simulink model "SPMSMSensorless"  (R2019b)
settings: Solver=VariableStepAuto  StartTime=0.0  StopTime=10  RelTol=1e-3
undefined symbols (not defined in the file): BmRated, DiscIntNeverNeededParam, etaFSO, etaPsiFSO, JmRated, K_dead, kFSO, KiId, KiIq, KiSpd, KpId, KpIq, kPsiFSO, KpSpd, LdRated, LqRated, OutCur_LowerLimit, OutCur_UpperLimit, OutSpd_LowerLimit, OutSpd_UpperLimit, PhiPMRated, Pn, RsRated, SetSpd_n, TsimCurLoop, TsimMotor, UdcRated, V_dead
libraries: simulink x3, eeTransforms x1, powerlib x1
(part 2 of 2)

== system SPMSMSensorless/PWM INT/FSO_RsInf/Clark Transformation4 ==
  U : Inport
  V : Inport  Port=2
  W : Inport  Port=3
  Add : Sum  Inputs=+--
  Add1 : Sum  Inputs=+-
  Gain : Gain  Gain=0.5
  Gain1 : Gain  Gain=0.5
  Gain2 : Gain  Gain=2/3
  Gain3 : Gain  Gain=2/3*0.86602540
  Alpha : Outport
  Beta : Outport  Port=2
  wires:
  Gain3/1 -> Beta/1
  Add1/1 -> Gain3/1
  Gain2/1 -> Alpha/1
  Add/1 -> Gain2/1
  U/1 -> Add/1
  Gain1/1 -> Add/3
  W/1 -> Gain1/1, Add1/2
  Gain/1 -> Add/2
  V/1 -> Gain/1, Add1/1

== system SPMSMSensorless/PWM INT/FSO_RsInf/PLL ==
  Eal : Inport
  Ebe : Inport  Port=2
  Add : Sum  Inputs=+-
  Cos : Trigonometry  Operator=cos
  Discrete-Time Integrator : DiscreteIntegrator  SampleTime=-1  ICPrevOutput=DiscIntNeverNeededParam  ICPrevScaledInput=DiscIntNeverNeededParam
  PID Controller : simulink/Continuous/PID Controller  Controller=PI  Form=Parallel  TimeDomain=Discrete-time  SampleTime=-1  IntegratorMethod=Forward Euler  FilterMethod=Forward Euler  ControllerParametersSource=internal  P=2*10*2*pi  I=(10*2*pi)^2  D=0  UseFilter=on  N=100  TunerSelectOption=Transfer Function Based (PID Tuner App)  InitialConditionSource=internal  InitialConditionForIntegrator=SetSpd_n*5/60*2*pi  InitialConditionForFilter=0  DifferentiatorICPrevScaledInput=0  ExternalReset=none  TrackingMode=off  Kt=1  LimitOutput=off  UpperSaturationLimit=inf  LowerSaturationLimit=-inf  LinearizeAsGain=on  AntiWindupMode=none  Kb=1  POutMin=[]  POutMax=[]  IOutMin=[]  IOutMax=[]  DOutMin=[]  DOutMax=[]  NOutMin=[]  NOutMax=[]  SumOutMin=[]  SumOutMax=[]  SaturationOutMin=[]  SaturationOutMax=[]  PParamMin=[]  PParamMax=[]  IParamMin=[]  IParamMax=[]  DParamMin=[]  DParamMax=[]  NParamMin=[]  NParamMax=[]  KbParamMin=[]  KbParamMax=[]  KtParamMin=[]  KtParamMax=[]  KbOutMin=[]  KbOutMax=[]  KtOutMin=[]  KtOutMax=[]  IntegratorOutMin=[]  IntegratorOutMax=[]  FilterOutMin=[]  FilterOutMax=[]  SumI1OutMin=[]  SumI1OutMax=[]  SumI2OutMin=[]  SumI2OutMax=[]  SumI3OutMin=[]  SumI3OutMax=[]  SumI4OutMin=[]  SumI4OutMax=[]  SumDOutMin=[]  SumDOutMax=[]  DifferentiatorOutMin=[]  DifferentiatorOutMax=[]  FilterDiffOutCoefMin=[]  FilterDiffOutCoefMax=[]  ReciprocalOutMin=[]  ReciprocalOutMax=[]  SumDenOutMin=[]  SumDenOutMax=[]  SumNumOutMin=[]  SumNumOutMax=[]  DivideOutMin=[]  DivideOutMax=[]  IntegratorContinuousStateAttributes=''  IntegratorStateMustResolveToSignalObject=off  IntegratorRTWStateStorageClass=Auto  FilterContinuousStateAttributes=''  FilterStateMustResolveToSignalObject=off  FilterRTWStateStorageClass=Auto  ParallelPVariant=InternalParameters  IdealPVariant=Disabled  IVariant=InternalParameters  DVariant=Disabled  IntegratorVariant=Discrete  SatVariant=Disabled  AWVariant=Passthrough  PCopyVariant=Disabled  TRVariant=Disabled  FdbkBlocksVariant=Forward  IdealPFdbkVariant=Disabled  SatFdbkVariant=Disabled  DerivativeFilterVariant=Disabled  NVariant=Disabled  NCopyVariant=Disabled_SignalSpec  FilterICVariant=Disabled  IntegratorICVariant=InternalICs  ExternalResetVariant=Disabled  TRSumVariant=Passthrough  SumFdbkVariant=Disabled  SumVariant=Sum_PI
  Product : Product
  Product1 : Product
  Sin : Trigonometry
  Unit Delay2 : UnitDelay  SampleTime=-1  HasFrameUpgradeWarning=on
  Unit Delay3 : UnitDelay  SampleTime=-1  HasFrameUpgradeWarning=on
  OmegaE : Outport
  ThetaE : Outport  Port=2
  wires:
  Sin/1 -> Product1/2
  Eal/1 -> Product/1
  Discrete-Time Integrator/1 -> ThetaE/1, Unit Delay3/1, Unit Delay2/1
  Unit Delay2/1 -> Cos/1
  Unit Delay3/1 -> Sin/1
  Product1/1 -> Add/2
  Product/1 -> Add/1
  Cos/1 -> Product/2
  Add/1 -> PID Controller/1
  Ebe/1 -> Product1/1
  PID Controller/1 -> Discrete-Time Integrator/1, OmegaE/1

== system SPMSMSensorless/PWM INT/FSO_RsInfPLL/Clark Transformation3 ==
  U : Inport
  V : Inport  Port=2
  W : Inport  Port=3
  Add : Sum  Inputs=+--
  Add1 : Sum  Inputs=+-
  Gain : Gain  Gain=0.5
  Gain1 : Gain  Gain=0.5
  Gain2 : Gain  Gain=2/3
  Gain3 : Gain  Gain=2/3*0.86602540
  Alpha : Outport
  Beta : Outport  Port=2
  wires:
  V/1 -> Add1/1, Gain/1
  Gain/1 -> Add/2
  W/1 -> Add1/2, Gain1/1
  Gain1/1 -> Add/3
  U/1 -> Add/1
  Add/1 -> Gain2/1
  Gain2/1 -> Alpha/1
  Add1/1 -> Gain3/1
  Gain3/1 -> Beta/1

== system SPMSMSensorless/PWM INT/FSO_RsInfPLL/Clark Transformation4 ==
  U : Inport
  V : Inport  Port=2
  W : Inport  Port=3
  Add : Sum  Inputs=+--
  Add1 : Sum  Inputs=+-
  Gain : Gain  Gain=0.5
  Gain1 : Gain  Gain=0.5
  Gain2 : Gain  Gain=2/3
  Gain3 : Gain  Gain=2/3*0.86602540
  Alpha : Outport
  Beta : Outport  Port=2
  wires:
  V/1 -> Add1/1, Gain/1
  Gain/1 -> Add/2
  W/1 -> Add1/2, Gain1/1
  Gain1/1 -> Add/3
  U/1 -> Add/1
  Add/1 -> Gain2/1
  Gain2/1 -> Alpha/1
  Add1/1 -> Gain3/1
  Gain3/1 -> Beta/1

== system SPMSMSensorless/PWM INT/FSO_RsInfPLL/LPF ==
  In1 : Inport
  Add1 : Sum
  Gain1 : Gain  Gain=1-0.1
  Gain3 : Gain  Gain=0.1
  Unit Delay1 : UnitDelay  SampleTime=-1  HasFrameUpgradeWarning=on
  Out1 : Outport
  wires:
  Add1/1 -> Out1/1, Unit Delay1/1
  Gain1/1 -> Add1/2
  Unit Delay1/1 -> Gain1/1
  Gain3/1 -> Add1/1
  In1/1 -> Gain3/1

== system SPMSMSensorless/PWM INT/FSO_RsInfPLL/PLL ==
  Eal : Inport
  Ebe : Inport  Port=2
  Add : Sum  Inputs=+-
  Cos : Trigonometry  Operator=cos
  Discrete-Time Integrator : DiscreteIntegrator  SampleTime=-1  ICPrevOutput=DiscIntNeverNeededParam  ICPrevScaledInput=DiscIntNeverNeededParam
  Gain1 : Gain  Gain=-1
  PID Controller : simulink/Continuous/PID Controller  Controller=PI  Form=Parallel  TimeDomain=Discrete-time  SampleTime=-1  IntegratorMethod=Forward Euler  FilterMethod=Forward Euler  ControllerParametersSource=internal  P=2*10*2*pi  I=(10*2*pi)^2  D=0  UseFilter=on  N=100  TunerSelectOption=Transfer Function Based (PID Tuner App)  InitialConditionSource=internal  InitialConditionForIntegrator=SetSpd_n*5/60*2*pi  InitialConditionForFilter=0  DifferentiatorICPrevScaledInput=0  ExternalReset=none  TrackingMode=off  Kt=1  LimitOutput=off  UpperSaturationLimit=inf  LowerSaturationLimit=-inf  LinearizeAsGain=on  AntiWindupMode=none  Kb=1  POutMin=[]  POutMax=[]  IOutMin=[]  IOutMax=[]  DOutMin=[]  DOutMax=[]  NOutMin=[]  NOutMax=[]  SumOutMin=[]  SumOutMax=[]  SaturationOutMin=[]  SaturationOutMax=[]  PParamMin=[]  PParamMax=[]  IParamMin=[]  IParamMax=[]  DParamMin=[]  DParamMax=[]  NParamMin=[]  NParamMax=[]  KbParamMin=[]  KbParamMax=[]  KtParamMin=[]  KtParamMax=[]  KbOutMin=[]  KbOutMax=[]  KtOutMin=[]  KtOutMax=[]  IntegratorOutMin=[]  IntegratorOutMax=[]  FilterOutMin=[]  FilterOutMax=[]  SumI1OutMin=[]  SumI1OutMax=[]  SumI2OutMin=[]  SumI2OutMax=[]  SumI3OutMin=[]  SumI3OutMax=[]  SumI4OutMin=[]  SumI4OutMax=[]  SumDOutMin=[]  SumDOutMax=[]  DifferentiatorOutMin=[]  DifferentiatorOutMax=[]  FilterDiffOutCoefMin=[]  FilterDiffOutCoefMax=[]  ReciprocalOutMin=[]  ReciprocalOutMax=[]  SumDenOutMin=[]  SumDenOutMax=[]  SumNumOutMin=[]  SumNumOutMax=[]  DivideOutMin=[]  DivideOutMax=[]  IntegratorContinuousStateAttributes=''  IntegratorStateMustResolveToSignalObject=off  IntegratorRTWStateStorageClass=Auto  FilterContinuousStateAttributes=''  FilterStateMustResolveToSignalObject=off  FilterRTWStateStorageClass=Auto  ParallelPVariant=InternalParameters  IdealPVariant=Disabled  IVariant=InternalParameters  DVariant=Disabled  IntegratorVariant=Discrete  SatVariant=Disabled  AWVariant=Passthrough  PCopyVariant=Disabled  TRVariant=Disabled  FdbkBlocksVariant=Forward  IdealPFdbkVariant=Disabled  SatFdbkVariant=Disabled  DerivativeFilterVariant=Disabled  NVariant=Disabled  NCopyVariant=Disabled_SignalSpec  FilterICVariant=Disabled  IntegratorICVariant=InternalICs  ExternalResetVariant=Disabled  TRSumVariant=Passthrough  SumFdbkVariant=Disabled  SumVariant=Sum_PI
  Product : Product
  Product1 : Product
  Sin : Trigonometry
  Unit Delay2 : UnitDelay  SampleTime=-1  HasFrameUpgradeWarning=on
  Unit Delay3 : UnitDelay  SampleTime=-1  HasFrameUpgradeWarning=on
  OmegaE : Outport
  ThetaE : Outport  Port=2
  wires:
  Sin/1 -> Product1/2
  Gain1/1 -> Product/1
  Discrete-Time Integrator/1 -> ThetaE/1, Unit Delay3/1, Unit Delay2/1
  Unit Delay2/1 -> Cos/1
  Unit Delay3/1 -> Sin/1
  Product1/1 -> Add/2
  Product/1 -> Add/1
  Cos/1 -> Product/2
  Add/1 -> PID Controller/1
  Ebe/1 -> Product1/1
  Eal/1 -> Gain1/1
  PID Controller/1 -> Discrete-Time Integrator/1, OmegaE/1

== system SPMSMSensorless/PWM INT/PsiFSO/Clark Transformation3 ==
  U : Inport
  V : Inport  Port=2
  W : Inport  Port=3
  Add : Sum  Inputs=+--
  Add1 : Sum  Inputs=+-
  Gain : Gain  Gain=0.5
  Gain1 : Gain  Gain=0.5
  Gain2 : Gain  Gain=2/3
  Gain3 : Gain  Gain=2/3*0.86602540
  Alpha : Outport
  Beta : Outport  Port=2
  wires:
  Gain3/1 -> Beta/1
  Add1/1 -> Gain3/1
  Gain2/1 -> Alpha/1
  Add/1 -> Gain2/1
  U/1 -> Add/1
  Gain1/1 -> Add/3
  W/1 -> Gain1/1, Add1/2
  Gain/1 -> Add/2
  V/1 -> Gain/1, Add1/1

== system SPMSMSensorless/PWM INT/PsiFSO/Clark Transformation4 ==
  U : Inport
  V : Inport  Port=2
  W : Inport  Port=3
  Add : Sum  Inputs=+--
  Add1 : Sum  Inputs=+-
  Gain : Gain  Gain=0.5
  Gain1 : Gain  Gain=0.5
  Gain2 : Gain  Gain=2/3
  Gain3 : Gain  Gain=2/3*0.86602540
  Alpha : Outport
  Beta : Outport  Port=2
  wires:
  Gain3/1 -> Beta/1
  Add1/1 -> Gain3/1
  Gain2/1 -> Alpha/1
  Add/1 -> Gain2/1
  U/1 -> Add/1
  Gain1/1 -> Add/3
  W/1 -> Gain1/1, Add1/2
  Gain/1 -> Add/2
  V/1 -> Gain/1, Add1/1

== system SPMSMSensorless/PWM INT/PsiFSORsAD/Clark Transformation3 ==
  U : Inport
  V : Inport  Port=2
  W : Inport  Port=3
  Add : Sum  Inputs=+--
  Add1 : Sum  Inputs=+-
  Gain : Gain  Gain=0.5
  Gain1 : Gain  Gain=0.5
  Gain2 : Gain  Gain=2/3
  Gain3 : Gain  Gain=2/3*0.86602540
  Alpha : Outport
  Beta : Outport  Port=2
  wires:
  V/1 -> Add1/1, Gain/1
  Gain/1 -> Add/2
  W/1 -> Add1/2, Gain1/1
  Gain1/1 -> Add/3
  U/1 -> Add/1
  Add/1 -> Gain2/1
  Gain2/1 -> Alpha/1
  Add1/1 -> Gain3/1
  Gain3/1 -> Beta/1

== system SPMSMSensorless/PWM INT/PsiFSORsAD/Clark Transformation4 ==
  U : Inport
  V : Inport  Port=2
  W : Inport  Port=3
  Add : Sum  Inputs=+--
  Add1 : Sum  Inputs=+-
  Gain : Gain  Gain=0.5
  Gain1 : Gain  Gain=0.5
  Gain2 : Gain  Gain=2/3
  Gain3 : Gain  Gain=2/3*0.86602540
  Alpha : Outport
  Beta : Outport  Port=2
  wires:
  V/1 -> Add1/1, Gain/1
  Gain/1 -> Add/2
  W/1 -> Add1/2, Gain1/1
  Gain1/1 -> Add/3
  U/1 -> Add/1
  Add/1 -> Gain2/1
  Gain2/1 -> Alpha/1
  Add1/1 -> Gain3/1
  Gain3/1 -> Beta/1

== system SPMSMSensorless/PWM INT/PsiFSORsInf/Clark Transformation3 ==
  U : Inport
  V : Inport  Port=2
  W : Inport  Port=3
  Add : Sum  Inputs=+--
  Add1 : Sum  Inputs=+-
  Gain : Gain  Gain=0.5
  Gain1 : Gain  Gain=0.5
  Gain2 : Gain  Gain=2/3
  Gain3 : Gain  Gain=2/3*0.86602540
  Alpha : Outport
  Beta : Outport  Port=2
  wires:
  V/1 -> Add1/1, Gain/1
  Gain/1 -> Add/2
  W/1 -> Add1/2, Gain1/1
  Gain1/1 -> Add/3
  U/1 -> Add/1
  Add/1 -> Gain2/1
  Gain2/1 -> Alpha/1
  Add1/1 -> Gain3/1
  Gain3/1 -> Beta/1

== system SPMSMSensorless/PWM INT/PsiFSORsInf/Clark Transformation4 ==
  U : Inport
  V : Inport  Port=2
  W : Inport  Port=3
  Add : Sum  Inputs=+--
  Add1 : Sum  Inputs=+-
  Gain : Gain  Gain=0.5
  Gain1 : Gain  Gain=0.5
  Gain2 : Gain  Gain=2/3
  Gain3 : Gain  Gain=2/3*0.86602540
  Alpha : Outport
  Beta : Outport  Port=2
  wires:
  V/1 -> Add1/1, Gain/1
  Gain/1 -> Add/2
  W/1 -> Add1/2, Gain1/1
  Gain1/1 -> Add/3
  U/1 -> Add/1
  Add/1 -> Gain2/1
  Gain2/1 -> Alpha/1
  Add1/1 -> Gain3/1
  Gain3/1 -> Beta/1

== system SPMSMSensorless/PWM INT/RealVoltageCompesation /Clark Transformation ==
  U : Inport
  V : Inport  Port=2
  W : Inport  Port=3
  Add : Sum  Inputs=+--
  Add1 : Sum  Inputs=+-
  Gain : Gain  Gain=0.5
  Gain1 : Gain  Gain=0.5
  Gain2 : Gain  Gain=2/3
  Gain3 : Gain  Gain=2/3*0.86602540
  Alpha : Outport
  Beta : Outport  Port=2
  wires:
  V/1 -> Add1/1, Gain/1
  Gain/1 -> Add/2
  W/1 -> Add1/2, Gain1/1
  Gain1/1 -> Add/3
  U/1 -> Add/1
  Add/1 -> Gain2/1
  Gain2/1 -> Alpha/1
  Add1/1 -> Gain3/1
  Gain3/1 -> Beta/1

== system SPMSMSensorless/PWM INT/RealVoltageCompesation /Park Transformation ==
  Alpha : Inport
  Beta : Inport  Port=2
  theta : Inport  Port=3
  Add : Sum
  Add1 : Sum  Inputs=+-
  Product{,1..3} (4 alike) : Product
  Sin : Trigonometry  OutputSignalType=real
  Sin1 : Trigonometry  Operator=cos  OutputSignalType=real
  D : Outport
  Q : Outport  Port=2
  wires:
  Product/1 -> Add/1
  Sin/1 -> Product3/2, Product1/2
  Product1/1 -> Add/2
  Add1/1 -> Q/1
  Sin1/1 -> Product2/2, Product/2
  Product2/1 -> Add1/1
  Alpha/1 -> Product3/1, Product/1
  Beta/1 -> Product2/1, Product1/1
  Product3/1 -> Add1/2
  Add/1 -> D/1
  theta/1 -> Sin/1, Sin1/1

== system SPMSMSensorless/PWM INT/RealVoltageCompesation /Park Transformation1 ==
  Alpha : Inport
  Beta : Inport  Port=2
  theta : Inport  Port=3
  Add : Sum
  Add1 : Sum  Inputs=+-
  Product{,1..3} (4 alike) : Product
  Sin : Trigonometry  OutputSignalType=real
  Sin1 : Trigonometry  Operator=cos  OutputSignalType=real
  D : Outport
  Q : Outport  Port=2
  wires:
  theta/1 -> Sin1/1, Sin/1
  Add/1 -> D/1
  Product3/1 -> Add1/2
  Beta/1 -> Product1/1, Product2/1
  Alpha/1 -> Product/1, Product3/1
  Product2/1 -> Add1/1
  Sin1/1 -> Product/2, Product2/2
  Add1/1 -> Q/1
  Product1/1 -> Add/2
  Sin/1 -> Product1/2, Product3/2
  Product/1 -> Add/1

== system SPMSMSensorless/PWM INT/SVPWM/Inverse Park Transformation ==
  D : Inport
  Q : Inport  Port=2
  theta : Inport  Port=3
  Product{,1..3} (4 alike) : Product  OutDataTypeStr=Inherit: Same as first input
  Sin : Trigonometry  OutputSignalType=real
  Sin1 : Trigonometry  Operator=cos  OutputSignalType=real
  Sum1 : Sum  Inputs=|++  OutDataTypeStr=Inherit: Same as first input
  Sum2 : Sum  Inputs=|+-  OutDataTypeStr=Inherit: Same as first input
  Alpha : Outport
  Beta : Outport  Port=2
  wires:
  Sin1/1 -> Product2/2, Product/2
  Sin/1 -> Product3/2, Product1/2
  Product3/1 -> Sum1/2
  Sum1/1 -> Beta/1
  D/1 -> Product3/1, Product/1
  Product2/1 -> Sum1/1
  Sum2/1 -> Alpha/1
  Product/1 -> Sum2/1
  Product1/1 -> Sum2/2
  Q/1 -> Product2/1, Product1/1
  theta/1 -> Sin/1, Sin1/1

== system SPMSMSensorless/PWM INT/SpdLoop/PI_Spd ==
  wm_Ref : Inport
  "wm_Fbk " : Inport  Port=2
  Add : Sum  Inputs=+-
  Add1 : Sum
  Discrete-Time Integrator : DiscreteIntegrator  InitialCondition=7.4  SampleTime=-1  LimitOutput=on  UpperSaturationLimit=30  LowerSaturationLimit=-30  ICPrevOutput=DiscIntNeverNeededParam  ICPrevScaledInput=DiscIntNeverNeededParam
  Gain : Gain  Gain=KpSpd
  Gain1 : Gain  Gain=KiSpd
  Saturation : Saturate  UpperLimit=OutSpd_UpperLimit  LowerLimit=OutSpd_LowerLimit
  PI_SpdOut : Outport
  wires:
  Gain/1 -> Add1/1
  Add1/1 -> Saturation/1
  "wm_Fbk "/1 -> Add/2
  Gain1/1 -> Discrete-Time Integrator/1
  wm_Ref/1 -> Add/1
  Add/1 -> Gain1/1, Gain/1
  Saturation/1 -> PI_SpdOut/1
  Discrete-Time Integrator/1 -> Add1/2

== matlab function SPMSMSensorless/MCU INT Trigger ==
  data: Clock input
  events: INT_ENABLE output FUNCTION_CALL_EVENT
function SYS_ENABLE(Clock)
    if(Clock == 0)
        INT_ENABLE();
    end
end

== matlab function SPMSMSensorless/PWM INT/RealVoltageCompesation /MATLAB Function1 ==
  data: I input; Uerror output; K input; Udead input
function Uerror = VSIComp(I,K,Udead)
Uerror = (2) * Udead * ((1)/((1) + exp(-K*I))-(0.5));
end

== matlab function SPMSMSensorless/PWM INT/MATLAB Function ==
  events: SPEED_ENABLE output FUNCTION_CALL_EVENT
function SpeedLoop()
    persistent Count;
    if isempty(Count)
        Count = 0;
    end
    
    Count = Count + 1;
    
    if(Count == 10)
        SPEED_ENABLE();
        Count = 0;
    end
end

== matlab function SPMSMSensorless/PWM INT/FSO/MATLAB Function2 ==
  data: Ual input; IalEst_Out output; Ube input; Ial input; Ibe input; SetSpd_n parameter; PhiPMRated parameter; Pn parameter; TsimCurLoop parameter; LqRated parameter; RsRated parameter; IbeEst_Out output; EalEst_Out output; EbeEst_Out output; kFSO parameter; etaFSO parameter; Theta_Out output; Omega_Out output; nRef input
function [IalEst_Out,IbeEst_Out,EalEst_Out,EbeEst_Out,Theta_Out,Omega_Out] = FSO(Ual,Ube,Ial,Ibe,SetSpd_n,PhiPMRated, Pn, TsimCurLoop, LqRated, RsRated,kFSO, etaFSO,nRef)
persistent IalEst IbeEst EalEst EbeEst OmegaEst ThetaEst;
if isempty(IalEst)
	IalEst = 0;
    IbeEst = 0;
    EalEst = -0.1;
    OmegaEst = SetSpd_n * Pn / 60 * 2 * pi;
    EbeEst = OmegaEst * PhiPMRated;
    ThetaEst = 0;
end
Ts = TsimCurLoop;
I = [1 0; 0  1;];
J = [0 -1; 1 0;];
i = [Ial,Ibe;]'; u = [Ual,Ube;]'; iEst = [IalEst,IbeEst;]'; eEst = [EalEst,EbeEst;]';
iTlide = iEst - i;
sgn = sign(iTlide);
RsFSO = RsRated;
LqFSO = LqRated * 0.8;

phi = 0.1;
if(iTlide(1) < phi && iTlide(1) > -phi)
    sgn(1) = iTlide(1)/phi;
end
if(iTlide(2) < phi && iTlide(2) > -phi)
    sgn(2) = iTlide(2)/phi;
end

iDot = - (RsFSO * I) * iEst + I * u - I * eEst + (kFSO * I) * sgn;
iDot = iDot./LqFSO;
iPre = iDot.* Ts + iEst;
IalEst = iPre(1); IbeEst = iPre(2);
IalEst_Out = IalEst; IbeEst_Out = IbeEst;

T = kFSO * [etaFSO,OmegaEst;-OmegaEst,etaFSO];
eDot = OmegaEst * J * eEst + T * sgn;
ePre = eEst + eDot .* Ts;
EalEst = ePre(1); EbeEst = ePre(2);
EalEst_Out = EalEst; EbeEst_Out = EbeEst;

ThetaPre = atan2(-EalEst * sign(OmegaEst),EbeEst * sign(OmegaEst));
% ThetaPre = atan2(-EalEst * OmegaEst,EbeEst * OmegaEst);
% ThetaPre = atan2(-EalEst,EbeEst);
Omega = (ThetaPre - ThetaEst);
if(Omega > pi)
    Omega = Omega - 2 * pi; 
elseif(Omega < -pi)
    Omega = Omega + 2 * pi;
end
Omega = Omega / Ts;
y = 0.999;
OmegaEst = OmegaEst * y + Omega * (1 - y);

ThetaEst = ThetaPre;
Theta_Out = ThetaEst;
Omega_Out = OmegaEst;

== matlab function SPMSMSensorless/PWM INT/RealVoltageCompesation /MATLAB Function2 ==
  data: I input; Uerror output; K input; Udead input
function Uerror = VSIComp(I,K,Udead)
Uerror = (2) * Udead * ((1)/((1) + exp(-K*I))-(0.5));
end

== matlab function SPMSMSensorless/PWM INT/SVPWM/MATLAB Function1 ==
  data: alpha input; ta output; beta input; tb output; tc output
function [ta,tb,tc] = SVPWM(alpha,beta)

temp1=beta;
temp2=0.5*beta+0.86603*alpha;
temp3=temp2-temp1;

VecSector=3;
if(temp2>0)
    VecSector=VecSector-1;
end
if(temp3>0)
    VecSector=VecSector-1;
end
if(temp1<0)
    VecSector=7-VecSector;
end

switch VecSector
    case 1
        ta=temp2;
        tb=temp1-temp3;
        tc=-temp2;
    case 2
        ta=temp3+temp2;
        tb=temp1;
        tc=-temp1;
    case 3
        ta=temp3;
        tb=-temp3;
        tc=-(temp1+temp2);
    case 4
        ta=temp2;
        tb=temp1-temp3;
        tc=-temp2;
    case 5
        ta=temp3+temp2;
        tb=temp1;
        tc=-temp1;
    case 6
        ta=temp3;
        tb=-temp3;
        tc=-(temp1+temp2);
    otherwise
        ta=(0.5);
        tb=(0.5);
        tc=(0.5);
end

== matlab function SPMSMSensorless/PWM INT/FSO/MATLAB Function1 ==
  data: ThetaEst input; ThetaError output; ThetaReal input
function ThetaError = Theta_Tilde(ThetaEst,ThetaReal)
ThetaError = ThetaEst - ThetaReal;
if(ThetaError < - pi)
    ThetaError = ThetaError + 2 * pi;
elseif(ThetaError > pi)
    ThetaError = ThetaError - 2 * pi;
end

== matlab function SPMSMSensorless/Motor/VSINonlinearity/MATLAB Function1 ==
  data: I input; U output; K input; Vdead input
function U = VSI_Nonlinearity(I,K,Vdead)
    U = Vdead*atan(I)/pi*2;
end

== matlab function SPMSMSensorless/Motor/VSINonlinearity/MATLAB Function2 ==
  data: I input; U output; K input; Vdead input
function U = VSI_Nonlinearity(I,K,Vdead)
    U = Vdead*atan(I)/pi*2;
end

== matlab function SPMSMSensorless/Motor/VSINonlinearity/MATLAB Function3 ==
  data: I input; U output; K input; Vdead input
function U = VSI_Nonlinearity(I,K,Vdead)
    U = Vdead*atan(I)/pi*2;
end

== matlab function SPMSMSensorless/PWM INT/FSO_RsInf/MATLAB Function3 ==
  data: ThetaEst input; ThetaError output; ThetaReal input
function ThetaError = Theta_Tilde(ThetaEst,ThetaReal)
ThetaError = ThetaEst - ThetaReal;
if(ThetaError < - pi)
    ThetaError = ThetaError + 2 * pi;
elseif(ThetaError > pi)
    ThetaError = ThetaError - 2 * pi;
end

== matlab function SPMSMSensorless/PWM INT/FSO_RsInf/MATLAB Function4 ==
  data: Ual input; IalEst_Out output; Ube input; Ial input; Ibe input; SetSpd_n parameter; PhiPMRated parameter; Pn parameter; TsimCurLoop parameter; LqRated parameter; RsRated parameter; IbeEst_Out output; EalEstInf_Out output; EbeEstInf_Out output; kFSO parameter; etaFSO parameter; Theta_Out output; Omega_Out output; Theta_OutInf output; nRef input; OmegaFbk input
function [IalEst_Out,IbeEst_Out,EalEstInf_Out,EbeEstInf_Out,Theta_Out,Omega_Out,Theta_OutInf] = FSO_RsInf(Ual,Ube,Ial,Ibe,SetSpd_n,PhiPMRated, Pn, TsimCurLoop, LqRated, RsRated,kFSO, etaFSO,nRef, OmegaFbk)
persistent IalEst IbeEst EalEst EbeEst OmegaEst ThetaEst;
if isempty(IalEst)
	IalEst = 0;
    IbeEst = 0;
    EalEst = -0.1;
    OmegaEst = SetSpd_n * Pn / 60 * 2 * pi;
    EbeEst = - OmegaEst * PhiPMRated;
    ThetaEst = 0;
end
Ts = TsimCurLoop;
I = [1 0; 0  1;];
J = [0 -1; 1 0;];
i = [Ial,Ibe;]'; u = [Ual,Ube;]'; iEst = [IalEst,IbeEst;]'; eEst = [EalEst,EbeEst;]';
iTlide = iEst - i;
sgn = sign(iTlide);
RsFSO = RsRated;
LqFSO = LqRated * 1.0;
RsInf = RsFSO * -1;

phi = 0.1;
if(iTlide(1) < phi && iTlide(1) > -phi)
    sgn(1) = iTlide(1)/phi;
end
if(iTlide(2) < phi && iTlide(2) > -phi)
    sgn(2) = iTlide(2)/phi;
end

iDot = - (RsInf * I) * iEst + I * u - I * eEst - (RsFSO * I - RsInf * I) * iEst + (kFSO * I) * sgn;
iDot = iDot./LqFSO;
iPre = iDot.* Ts + iEst;
IalEst = iPre(1); IbeEst = iPre(2);
IalEst_Out = IalEst; IbeEst_Out = IbeEst;

sign_omega = sign(OmegaFbk);
% sign_omega = sign(1);
if sign_omega == 0
    sign_omega = 1;
end

% T = kFSO * [etaFSO,OmegaEst;-OmegaEst,etaFSO];
T = kFSO * [etaFSO,OmegaFbk;-OmegaFbk,etaFSO];
% eDot = OmegaEst * J * eEst + T * sgn;
eDot = OmegaFbk * J * eEst + T * sgn;
ePre = eEst + eDot .* Ts;
EalEst = ePre(1); EbeEst = ePre(2);

eEstInf = eEst + (RsFSO * I - RsInf * I) * iEst * sign_omega;
EalEstInf = eEstInf(1);
EbeEstInf = eEstInf(2);

EalEstInf_Out = EalEstInf; EbeEstInf_Out = EbeEstInf;

ThetaPreInf = atan2(-EalEstInf * sign(sign_omega),EbeEstInf * sign(sign_omega));

% ThetaPreInf = atan2(-EalEst,EbeEst);

Omega = (ThetaPreInf - ThetaEst);
if(Omega > pi)
    Omega = Omega - 2 * pi; 
elseif(Omega < -pi)
    Omega = Omega + 2 * pi;
end
Omega = Omega / Ts;
y = 0.999;
OmegaEst = OmegaEst * y + Omega * (1 - y);
% OmegaEst = nRef * Pn / 60 * 2 * pi;

ThetaEst = ThetaPreInf;
Theta_Out = ThetaEst;
Theta_OutInf = ThetaPreInf;
Omega_Out = OmegaEst;

== matlab function SPMSMSensorless/PWM INT/FSO_Flux_SpdOb/MATLAB Function1 ==
  data: ThetaEst input; ThetaError output; ThetaReal input
function ThetaError = Theta_Tilde(ThetaEst,ThetaReal)
ThetaError = ThetaEst - ThetaReal;
if(ThetaError < - pi)
    ThetaError = ThetaError + 2 * pi;
elseif(ThetaError > pi)
    ThetaError = ThetaError - 2 * pi;
end

== matlab function SPMSMSensorless/PWM INT/FSO_Flux_SpdOb/MATLAB Function2 ==
  data: Ual input; IalEst_Out output; Ube input; Ial input; Ibe input; SetSpd_n parameter; PhiPMRated parameter; Pn parameter; TsimCurLoop parameter; LqRated parameter; RsRated parameter; IbeEst_Out output; PsialEst_Out output; PsibeEst_Out output; kFSO parameter; etaFSO parameter; Theta_Out output; Omega_Out output; nRef input
function [IalEst_Out,IbeEst_Out,PsialEst_Out,PsibeEst_Out,Theta_Out,Omega_Out] = FSO(Ual,Ube,Ial,Ibe,SetSpd_n,PhiPMRated, Pn, TsimCurLoop, LqRated, RsRated,kFSO, etaFSO,nRef)
persistent IalEst IbeEst PsialEst PsibeEst OmegaEst ThetaEst;
if isempty(IalEst)
	IalEst = 0;
    IbeEst = 0;
    PsialEst = PhiPMRated;
    OmegaEst = SetSpd_n * Pn / 60 * 2 * pi;
    PsibeEst = 0;
    ThetaEst = 0;
end
Ts = TsimCurLoop;
I = [1 0; 0  1;];
J = [0 -1; 1 0;];
i = [Ial,Ibe;]'; u = [Ual,Ube;]'; iEst = [IalEst,IbeEst;]'; PsiEst = [PsialEst,PsibeEst;]';
iTlide = iEst - i;
sgn = sign(iTlide);
RsFSO = RsRated;
LqFSO = LqRated;

phi = 0.1;
if(iTlide(1) < phi && iTlide(1) > -phi)
    sgn(1) = iTlide(1)/phi;
end
if(iTlide(2) < phi && iTlide(2) > -phi)
    sgn(2) = iTlide(2)/phi;
end
h1 = -20;
h2 = -1;
h3 = (h1/2)^2 * 3e-3;
h4 = -h1 * 3e-3;
iDot = - (RsFSO * I) * i + I * u - OmegaEst * J * PsiEst + (h1 * I + h2 * J) * iTlide;
iDot = iDot./LqFSO;
iPre = iDot.* Ts + iEst;
IalEst = iPre(1); IbeEst = iPre(2);
IalEst_Out = IalEst; IbeEst_Out = IbeEst;

T = kFSO * [etaFSO,OmegaEst;-OmegaEst,etaFSO];
PsiDot = OmegaEst * J * PsiEst +  + (h3 * I + h4 * J) * iTlide;
PsiPre = PsiEst + PsiDot .* Ts;
PsialEst = PsiPre(1); PsibeEst = PsiPre(2);
PsialEst_Out = PsialEst; PsibeEst_Out = PsibeEst;

ThetaPre = atan2(-PsialEst/sign(nRef),PsibeEst/sign(nRef));

Ki = 10;
% Kp = 0.1;
OmegaEstDot = iTlide' * J * PsiEst;
OmegaEst = OmegaEst + OmegaEstDot * Ts * Ki;

ThetaEst = ThetaPre;
Theta_Out = ThetaEst;
Omega_Out = OmegaEst;

== matlab function SPMSMSensorless/PWM INT/FSO_RsInfPLL/MATLAB Function3 ==
  data: ThetaEst input; ThetaError output; ThetaReal input
function ThetaError = Theta_Tilde(ThetaEst,ThetaReal)
ThetaError = ThetaEst - ThetaReal;
if(ThetaError < - pi)
    ThetaError = ThetaError + 2 * pi;
elseif(ThetaError > pi)
    ThetaError = ThetaError - 2 * pi;
end

== matlab function SPMSMSensorless/PWM INT/FSO_RsInfPLL/MATLAB Function4 ==
  data: Ual input; IalEst_Out output; Ube input; Ial input; Ibe input; SetSpd_n parameter; PhiPMRated parameter; Pn parameter; TsimCurLoop parameter; LqRated parameter; RsRated parameter; IbeEst_Out output; EalEstInf_Out output; EbeEstInf_Out output; kFSO parameter; etaFSO parameter; nRef input; OmegaFbk input; OmegaEst input
function [IalEst_Out,IbeEst_Out,EalEstInf_Out,EbeEstInf_Out] = FSO_RsInfPLL(Ual,Ube,Ial,Ibe,SetSpd_n,PhiPMRated, Pn, TsimCurLoop, LqRated, RsRated,kFSO, etaFSO,nRef, OmegaFbk,OmegaEst)
persistent IalEst IbeEst EalEst EbeEst ThetaEst;
if isempty(IalEst)
	IalEst = 0;
    IbeEst = 0;
    EalEst = -0.1;
    EbeEst = - OmegaEst * PhiPMRated;
end
Ts = TsimCurLoop;
I = [1 0; 0  1;];
J = [0 -1; 1 0;];
i = [Ial,Ibe;]'; u = [Ual,Ube;]'; iEst = [IalEst,IbeEst;]'; eEst = [EalEst,EbeEst;]';
iTlide = iEst - i;
sgn = sign(iTlide);
RsFSO = RsRated;
LqFSO = LqRated;
RsInf = RsFSO * -0.5;

phi = 0.1;
if(iTlide(1) < phi && iTlide(1) > -phi)
    sgn(1) = iTlide(1)/phi;
end
if(iTlide(2) < phi && iTlide(2) > -phi)
    sgn(2) = iTlide(2)/phi;
end

iDot = - (RsInf * I) * iEst + I * u - I * eEst - (RsFSO * I - RsInf * I) * iEst + (kFSO * I) * sgn;
iDot = iDot./LqFSO;
iPre = iDot.* Ts + iEst;
IalEst = iPre(1); IbeEst = iPre(2);
IalEst_Out = IalEst; IbeEst_Out = IbeEst;

sign_omega = sign(OmegaEst);
if sign_omega == 0
    sign_omega = 1;
end

% T = kFSO * [etaFSO,OmegaEst;-OmegaEst,etaFSO];
T = kFSO * [etaFSO,OmegaFbk;-OmegaFbk,etaFSO];
eDot = OmegaEst * J * eEst + T * sgn;
% eDot = OmegaFbk * J * eEst + T * sgn;
ePre = eEst + eDot .* Ts;
EalEst = ePre(1); EbeEst = ePre(2);

eEstInf = eEst + (RsFSO * I - RsInf * I) * iEst;
EalEstInf = eEstInf(1) * sign(OmegaFbk);
EbeEstInf = eEstInf(2) * sign(OmegaFbk);

EalEstInf_Out = EalEstInf; EbeEstInf_Out = EbeEstInf;

== matlab function SPMSMSensorless/PWM INT/PsiFSO/MATLAB Function3 ==
  data: ThetaEst input; ThetaError output; ThetaReal input
function ThetaError = Theta_Tilde(ThetaEst,ThetaReal)
ThetaError = ThetaEst - ThetaReal;
if(ThetaError < - pi)
    ThetaError = ThetaError + 2 * pi;
elseif(ThetaError > pi)
    ThetaError = ThetaError - 2 * pi;
end

== matlab function SPMSMSensorless/PWM INT/PsiFSO/MATLAB Function4 ==
  data: Ual input; IalEst_Out output; Ube input; Ial input; Ibe input; SetSpd_n parameter; PhiPMRated parameter; Pn parameter; TsimCurLoop parameter; LqRated parameter; RsRated parameter; IbeEst_Out output; PsialEst_Out output; PsibeEst_Out output; kPsiFSO parameter; etaPsiFSO parameter; nRef input; OmegaFbk input; ThetaEst_Out output; OmegaEst_Out output
function [IalEst_Out,IbeEst_Out,PsialEst_Out,PsibeEst_Out,ThetaEst_Out,OmegaEst_Out] = PsiFSO(Ual,Ube,Ial,Ibe,SetSpd_n,PhiPMRated, Pn, TsimCurLoop, LqRated, RsRated,kPsiFSO, etaPsiFSO,nRef, OmegaFbk)
persistent IalEst IbeEst PsialEst PsibeEst ThetaEst OmegaEst;
if isempty(IalEst)
	IalEst = 0;
    IbeEst = 0;
    PsialEst = PhiPMRated;
    PsibeEst = 0;
    ThetaEst = 0;
    OmegaEst = SetSpd_n * Pn / 60 * 2 * pi;
end
Ts = TsimCurLoop;
I = [1 0; 0  1;];
J = [0 -1; 1 0;];
i = [Ial,Ibe;]'; u = [Ual,Ube;]'; iEst = [IalEst,IbeEst;]'; PsiEst = [PsialEst,PsibeEst;]';
iTlide = iEst - i;
sgn = sign(iTlide);
RsFSO = RsRated * 1.0;
LqFSO = LqRated * 1.0;

phi = 0.1;
if(iTlide(1) < phi && iTlide(1) > -phi)
    sgn(1) = iTlide(1)/phi;
end
if(iTlide(2) < phi && iTlide(2) > -phi)
    sgn(2) = iTlide(2)/phi;
end

iDot = - (RsFSO * I) * iEst + I * u - OmegaEst * J * PsiEst + (kPsiFSO * I) * sgn;
iDot = iDot./LqFSO;
iPre = iDot.* Ts + iEst;
IalEst = iPre(1); IbeEst = iPre(2);
IalEst_Out = IalEst; IbeEst_Out = IbeEst;

T =  - kPsiFSO * I + etaPsiFSO * J * OmegaEst / (abs(SetSpd_n) * Pn / 60 * 2 * pi);
PsiDot = OmegaEst * J * PsiEst + T * sgn;
PsiPre = PsiEst + PsiDot .* Ts;
% if(PsiPre(1) > 0.2)
%     PsiPre(1) = 0.2;
% elseif(PsiPre(1) < -0.2)
%     PsiPre(1) = -0.2;
% end
% 
% if(PsiPre(2) > 0.2)
%     PsiPre(2) = 0.2;
% elseif(PsiPre(2) < -0.2)
%     PsiPre(2) = -0.2;
% end
PsialEst = PsiPre(1); PsibeEst = PsiPre(2);
PsialEst_Out = PsialEst;
PsibeEst_Out = PsibeEst;


ThetaPre = atan2(PsibeEst,PsialEst);

OmegaPre = (ThetaPre - ThetaEst);
if(OmegaPre > pi)
    OmegaPre = OmegaPre - 2 * pi; 
elseif(OmegaPre < -pi)
    OmegaPre = OmegaPre + 2 * pi;
end
y = 0.1;
OmegaEst = OmegaPre/Ts * y + OmegaEst * (1 - y);
ThetaEst = ThetaPre;

ThetaEst_Out = ThetaEst;
OmegaEst_Out = OmegaEst;

== matlab function SPMSMSensorless/PWM INT/PsiFSORsInf/MATLAB Function3 ==
  data: ThetaEst input; ThetaError output; ThetaReal input
function ThetaError = Theta_Tilde(ThetaEst,ThetaReal)
ThetaError = ThetaEst - ThetaReal;
if(ThetaError < - pi)
    ThetaError = ThetaError + 2 * pi;
elseif(ThetaError > pi)
    ThetaError = ThetaError - 2 * pi;
end

== matlab function SPMSMSensorless/PWM INT/PsiFSORsInf/MATLAB Function4 ==
  data: Ual input; IalEst_Out output; Ube input; Ial input; Ibe input; SetSpd_n parameter; PhiPMRated parameter; Pn parameter; TsimCurLoop parameter; LqRated parameter; RsRated parameter; IbeEst_Out output; PsialEst_Out output; PsibeEst_Out output; kPsiFSO parameter; etaPsiFSO parameter; nRef input; OmegaFbk input; ThetaEst_Out output; OmegaEst_Out output
function [IalEst_Out,IbeEst_Out,PsialEst_Out,PsibeEst_Out,ThetaEst_Out,OmegaEst_Out] = PsiFSO(Ual,Ube,Ial,Ibe,SetSpd_n,PhiPMRated, Pn, TsimCurLoop, LqRated, RsRated,kPsiFSO, etaPsiFSO,nRef, OmegaFbk)
persistent IalEst IbeEst PsialEst PsibeEst ThetaEst OmegaEst;
if isempty(IalEst)
	IalEst = 0;
    IbeEst = 0;
    PsialEst = PhiPMRated;
    PsibeEst = 0;
    ThetaEst = 0;
    OmegaEst = SetSpd_n * Pn / 60 * 2 * pi;
end
Ts = TsimCurLoop;
I = [1 0; 0  1;];
J = [0 -1; 1 0;];
i = [Ial,Ibe;]'; u = [Ual,Ube;]'; iEst = [IalEst,IbeEst;]'; PsiEst = [PsialEst,PsibeEst;]';
iTlide = iEst - i;
sgn = sign(iTlide);
RsFSO = RsRated;
LqFSO = LqRated * 1.0;
RsInf = RsFSO * -2.5;

phi = 0.1;
if(iTlide(1) < phi && iTlide(1) > -phi)
    sgn(1) = iTlide(1)/phi;
end
if(iTlide(2) < phi && iTlide(2) > -phi)
    sgn(2) = iTlide(2)/phi;
end

iDot = - (RsInf * I) * iEst + I * u - (OmegaEst - (RsInf - RsFSO) * sqrt(Ial ^ 2 + Ibe ^ 2) / sqrt(PsialEst^2 + PsibeEst^2)) * J * PsiEst + (kPsiFSO * I) * sgn;
iDot = iDot./LqFSO;
iPre = iDot.* Ts + iEst;
IalEst = iPre(1); IbeEst = iPre(2);
IalEst_Out = IalEst; IbeEst_Out = IbeEst;

T =  - kPsiFSO * I + etaPsiFSO * (OmegaEst / (abs(SetSpd_n) * Pn / 60 * 2 * pi)) * J;
PsiDot = OmegaEst * J * PsiEst + T * sgn;
PsiPre = PsiEst + PsiDot .* Ts;
PsialEst = PsiPre(1); PsibeEst = PsiPre(2);
% PsiPreRsInf = PsiPre - J * (RsInf - RsFSO) * i ./ (nRef * Pn / 60 * 2 * pi);
PsiPreRsInf = PsiPre;
PsialEst_Out = PsiPreRsInf(1);
PsibeEst_Out = PsiPreRsInf(2);


ThetaPre = atan2(PsibeEst_Out,PsialEst_Out);

OmegaPre = (ThetaPre - ThetaEst);
if(OmegaPre > pi)
    OmegaPre = OmegaPre - 2 * pi; 
elseif(OmegaPre < -pi)
    OmegaPre = OmegaPre + 2 * pi;
end
y = 0.01;
OmegaEst = OmegaPre/Ts * y + OmegaEst * (1 - y);
ThetaEst = ThetaPre;

ThetaEst_Out = ThetaEst;
OmegaEst_Out = OmegaEst;

== matlab function SPMSMSensorless/PWM INT/PsiFSORsAD/MATLAB Function3 ==
  data: ThetaEst input; ThetaError output; ThetaReal input
function ThetaError = Theta_Tilde(ThetaEst,ThetaReal)
ThetaError = ThetaEst - ThetaReal;
if(ThetaError < - pi)
    ThetaError = ThetaError + 2 * pi;
elseif(ThetaError > pi)
    ThetaError = ThetaError - 2 * pi;
end

== matlab function SPMSMSensorless/PWM INT/PsiFSORsAD/MATLAB Function4 ==
  data: Ual input; IalEst_Out output; Ube input; Ial input; Ibe input; SetSpd_n parameter; PhiPMRated parameter; Pn parameter; TsimCurLoop parameter; LqRated parameter; RsRated parameter; IbeEst_Out output; PsialEst_Out output; PsibeEst_Out output; kPsiFSO parameter; etaPsiFSO parameter; nRef input; OmegaFbk input; ThetaEst_Out output; OmegaEst_Out output; RsOut output
function [IalEst_Out,IbeEst_Out,PsialEst_Out,PsibeEst_Out,ThetaEst_Out,OmegaEst_Out,RsOut] = PsiFSO(Ual,Ube,Ial,Ibe,SetSpd_n,PhiPMRated, Pn, TsimCurLoop, LqRated, RsRated,kPsiFSO, etaPsiFSO,nRef, OmegaFbk)
persistent IalEst IbeEst PsialEst PsibeEst ThetaEst OmegaEst RsEst;
if isempty(IalEst)
	IalEst = 0;
    IbeEst = 0;
    PsialEst = PhiPMRated;
    RsEst = RsRated * 0.8;
    PsibeEst = 0;
    ThetaEst = 0;
    OmegaEst = SetSpd_n * Pn / 60 * 2 * pi;
end
Ts = TsimCurLoop;
I = [1 0; 0  1;];
J = [0 -1; 1 0;];
i = [Ial,Ibe;]'; u = [Ual,Ube;]'; iEst = [IalEst,IbeEst;]'; PsiEst = [PsialEst,PsibeEst;]';
iTlide = iEst - i;
sgn = sign(iTlide);
RsFSO = RsRated * 1.0;
LqFSO = LqRated * 1.0;

phi = 0.1;
if(iTlide(1) < phi && iTlide(1) > -phi)
    sgn(1) = iTlide(1)/phi;
end
if(iTlide(2) < phi && iTlide(2) > -phi)
    sgn(2) = iTlide(2)/phi;
end

iDot = - (RsEst * I) * iEst + I * u - OmegaEst * J * PsiEst + (kPsiFSO * I) * sgn;
iDot = iDot./LqFSO;
iPre = iDot.* Ts + iEst;
IalEst = iPre(1); IbeEst = iPre(2);
IalEst_Out = IalEst; IbeEst_Out = IbeEst;

T =  - kPsiFSO * I + etaPsiFSO * J * OmegaEst / (abs(SetSpd_n) * Pn / 60 * 2 * pi);
PsiDot = OmegaEst * J * PsiEst + T * sgn;
PsiPre = PsiEst + PsiDot .* Ts;
% if(PsiPre(1) > 0.2)
%     PsiPre(1) = 0.2;
% elseif(PsiPre(1) < -0.2)
%     PsiPre(1) = -0.2;
% end
% 
% if(PsiPre(2) > 0.2)
%     PsiPre(2) = 0.2;
% elseif(PsiPre(2) < -0.2)
%     PsiPre(2) = -0.2;
% end
PsialEst = PsiPre(1); PsibeEst = PsiPre(2);
PsialEst_Out = PsialEst;
PsibeEst_Out = PsibeEst;
Psidm = sqrt(PsialEst^2 + PsibeEst^2);
RsEst = RsEst - (PhiPMRated - Psidm) * Ts * 100;


ThetaPre = atan2(PsibeEst,PsialEst);

OmegaPre = (ThetaPre - ThetaEst);
if(OmegaPre > pi)
    OmegaPre = OmegaPre - 2 * pi; 
elseif(OmegaPre < -pi)
    OmegaPre = OmegaPre + 2 * pi;
end
y = 0.1;
OmegaEst = OmegaPre/Ts * y + OmegaEst * (1 - y);
ThetaEst = ThetaPre;
RsOut = RsEst;
ThetaEst_Out = ThetaEst;
OmegaEst_Out = OmegaEst;

== matlab function SPMSMSensorless/PWM INT/FSOLqInf/MATLAB Function1 ==
  data: ThetaEst input; ThetaError output; ThetaReal input
function ThetaError = Theta_Tilde(ThetaEst,ThetaReal)
ThetaError = ThetaEst - ThetaReal;
if(ThetaError < - pi)
    ThetaError = ThetaError + 2 * pi;
elseif(ThetaError > pi)
    ThetaError = ThetaError - 2 * pi;
end

== matlab function SPMSMSensorless/PWM INT/FSOLqInf/MATLAB Function2 ==
  data: Ual input; IalEst_Out output; Ube input; Ial input; Ibe input; SetSpd_n parameter; PhiPMRated parameter; Pn parameter; TsimCurLoop parameter; LqRated parameter; RsRated parameter; IbeEst_Out output; EalEst_Out output; EbeEst_Out output; kFSO parameter; etaFSO parameter; Theta_Out output; Omega_Out output; nRef input
function [IalEst_Out,IbeEst_Out,EalEst_Out,EbeEst_Out,Theta_Out,Omega_Out] = FSO(Ual,Ube,Ial,Ibe,SetSpd_n,PhiPMRated, Pn, TsimCurLoop, LqRated, RsRated,kFSO, etaFSO,nRef)
persistent IalEst IbeEst EalEst EbeEst OmegaEst ThetaEst;
if isempty(IalEst)
	IalEst = 0;
    IbeEst = 0;
    EalEst = -0.1;
    OmegaEst = SetSpd_n * Pn / 60 * 2 * pi;
    EbeEst = OmegaEst * PhiPMRated;
    ThetaEst = 0;
end
Ts = TsimCurLoop;
I = [1 0; 0  1;];
J = [0 -1; 1 0;];
i = [Ial,Ibe;]'; u = [Ual,Ube;]'; iEst = [IalEst,IbeEst;]'; eEst = [EalEst,EbeEst;]';
iTlide = iEst - i;
sgn = sign(iTlide);
RsFSO = RsRated;
LqFSO = LqRated * 0.8;
LqInf = LqFSO * 200.0;

phi = 0.1;
if(iTlide(1) < phi && iTlide(1) > -phi)
    sgn(1) = iTlide(1)/phi;
end
if(iTlide(2) < phi && iTlide(2) > -phi)
    sgn(2) = iTlide(2)/phi;
end

iDot = - (RsFSO * I) * iEst + I * u - I * eEst + (kFSO * I) * sgn;
iDot = iDot./LqFSO;
iPre = iDot.* Ts + iEst;
IalEst = iPre(1); IbeEst = iPre(2);
IalEst_Out = IalEst; IbeEst_Out = IbeEst;

T = kFSO * [etaFSO,OmegaEst;-OmegaEst,etaFSO];
eDot = OmegaEst * J * eEst + T * sgn;
ePre = eEst + eDot .* Ts;
EalEst = ePre(1); EbeEst = ePre(2);

ePreInf = ePre + (LqFSO - LqInf) * J * (SetSpd_n * Pn / 60 * 2 * pi) * iEst;
EalEst_Out = ePreInf(1); EbeEst_Out = ePreInf(2);

% ThetaPre = atan2(-EalEst * sign(OmegaEst),EbeEst * sign(OmegaEst));
% ThetaPre = atan2(-EalEst * OmegaEst,EbeEst * OmegaEst);
ThetaPre = atan2(EbeEst_Out,EalEst_Out);
Omega = (ThetaPre - ThetaEst);
if(Omega > pi)
    Omega = Omega - 2 * pi; 
elseif(Omega < -pi)
    Omega = Omega + 2 * pi;
end
Omega = Omega / Ts;
y = 0.999;
OmegaEst = OmegaEst * y + Omega * (1 - y);

ThetaEst = ThetaPre;
Theta_Out = ThetaEst;
Omega_Out = OmegaEst;

== matlab function SPMSMSensorless/PWM INT/FSO_RsInf/MATLAB Function ==
  data: I input; Uerror output; K input; Udead input
function Uerror = VSIComp(I,K,Udead)
Uerror = (2) * Udead * ((1)/((1) + exp(-K*I))-(0.5));
end

== matlab function SPMSMSensorless/PWM INT/RealVoltageCompesation /MATLAB Function ==
  data: I input; Uerror output; K input; Udead input
function Uerror = VSIComp(I,K,Udead)
Uerror = (2) * Udead * ((1)/((1) + exp(-K*I))-(0.5));
end

== matlab function SPMSMSensorless/PWM INT/FSO_RsInf/MATLAB Function1 ==
  data: I input; Uerror output; K input; Udead input
function Uerror = VSIComp(I,K,Udead)
Uerror = (2) * Udead * ((1)/((1) + exp(-K*I))-(0.5));
end

== matlab function SPMSMSensorless/PWM INT/FSO_RsInf/MATLAB Function2 ==
  data: I input; Uerror output; K input; Udead input
function Uerror = VSIComp(I,K,Udead)
Uerror = (2) * Udead * ((1)/((1) + exp(-K*I))-(0.5));
end
